simulink model "a4_block"  (R2019b)
settings: Solver=VariableStepAuto  StartTime=0.0  StopTime=500  RelTol=1e-3
settings Model: Creator=sourabh  LastModifiedBy=sourabh
settings DataIOCC: ReturnWorkspaceOutputs=off

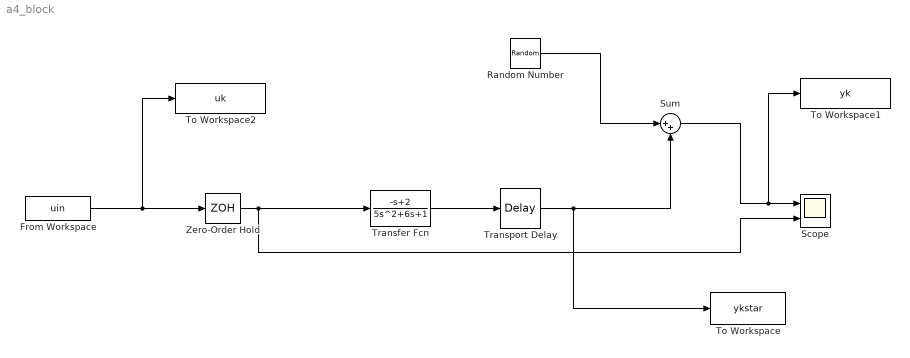
== system a4_block ==
  From Workspace : FromWorkspace  VariableName=uin  SampleTime=0
  Random Number : RandomNumber  Variance=0.1  SampleTime=0.1
  Scope : Scope  NumInputPorts=2
  Sum : Sum  Inputs=|++
  To Workspace : ToWorkspace  VariableName=ykstar  SampleTime=-1
  To Workspace1 : ToWorkspace  VariableName=yk  SampleTime=-1
  To Workspace2 : ToWorkspace  VariableName=uk  SampleTime=-1
  Transfer Fcn : TransferFcn  Numerator=[-1 2]  Denominator=[5 6 1]
  Transport Delay : TransportDelay  DelayTime=3
  Zero-Order Hold : ZeroOrderHold  SampleTime=-1
  wires:
  From Workspace/1 -> To Workspace2/1, Zero-Order Hold/1
  Zero-Order Hold/1 -> Scope/2, Transfer Fcn/1
  Transfer Fcn/1 -> Transport Delay/1
  Transport Delay/1 -> To Workspace/1, Sum/2
  Random Number/1 -> Sum/1
  Sum/1 -> To Workspace1/1, Scope/1
